simulink model "Quadrotor_model"  (R2020b)
settings: Solver=VariableStepAuto  StartTime=0.0  StopTime=10  RelTol=1e-3
model workspace (MAT data in the model file):
  Kheight = 1
  Kpitch = 1
  Kroll = 1
  Kyaw = 1
  pitch_dot_0 = 0
  roll_0 = 0
  roll_dot_0 = 0
  yaw_0 = 0
  yaw_dot_0 = 0
undefined symbols (not defined in the file or in its folder): pitch_0
libraries: pid_lib x4, simulink x1
settings Model: Creator=kike  LastModifiedBy=kike

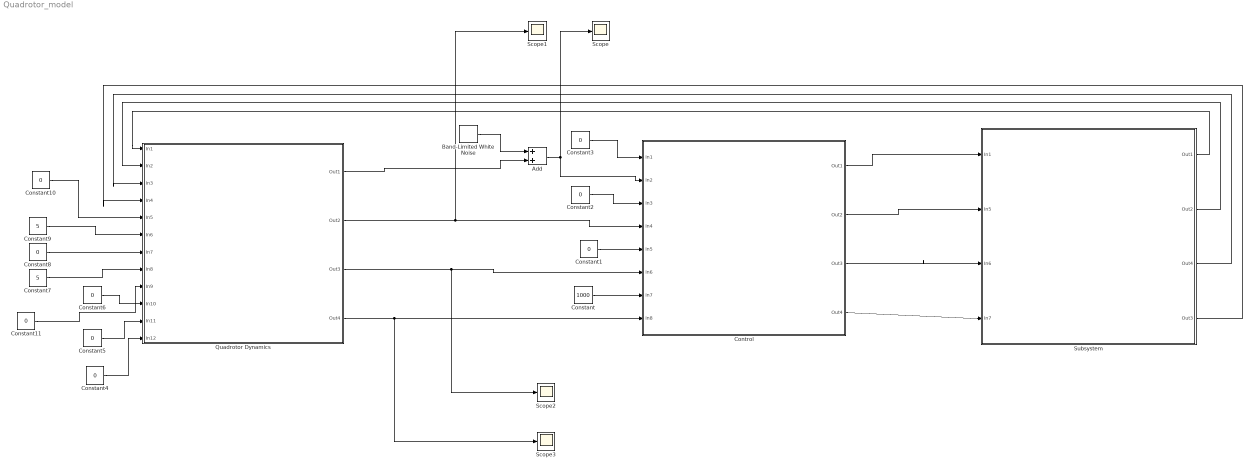
== system Quadrotor_model ==
  Add : Sum
  Band-Limited White Noise : simulink/Sources/Band-Limited White Noise  Cov=0  Ts=0.01  seed=[23341]
  Constant : Constant  Value=1000
  Constant{1..6,8,10..11} (9 alike) : Constant  Value=0
  Constant7 : Constant  Value=5
  Constant9 : Constant  Value=5
  Control : Subsystem
  Quadrotor Dynamics : Subsystem  Description=Quadrotor dynamics
  Scope{,1..3} (4 alike) : Scope
  Subsystem : Subsystem
  wires:
  Add/1 -> Scope/1, Control/2(In2)
  Quadrotor Dynamics/2(Out2) -> Scope1/1, Control/4(In4)
  Quadrotor Dynamics/3(Out3) -> Scope2/1, Control/6(In6)
  Quadrotor Dynamics/4(Out4) -> Scope3/1, Control/8(In8)
  Constant/1 -> Control/7(In7)
  Constant1/1 -> Control/5(In5)
  Constant2/1 -> Control/3(In3)
  Constant3/1 -> Control/1(In1)
  Constant4/1 -> Quadrotor Dynamics/12(In12)
  Constant5/1 -> Quadrotor Dynamics/11(In11)
  Constant6/1 -> Quadrotor Dynamics/10(In10)
  Constant7/1 -> Quadrotor Dynamics/8(In8)
  Constant8/1 -> Quadrotor Dynamics/7(In7)
  Constant9/1 -> Quadrotor Dynamics/6(In6)
  Constant10/1 -> Quadrotor Dynamics/5(In5)
  Constant11/1 -> Quadrotor Dynamics/9(In9)
  Control/1(Out1) -> Subsystem/1(In1)
  Control/2(Out2) -> Subsystem/2(In5)
  Control/3(Out3) -> Subsystem/3(In6)
  Control/4(Out4) -> Subsystem/4(In7)
  Subsystem/1(Out1) -> Quadrotor Dynamics/1(In1)
  Subsystem/2(Out2) -> Quadrotor Dynamics/2(In2)
  Subsystem/3(Out4) -> Quadrotor Dynamics/3(In3)
  Subsystem/4(Out3) -> Quadrotor Dynamics/4(In4)
  Band-Limited White Noise/1 -> Add/1
  Quadrotor Dynamics/1(Out1) -> Add/2

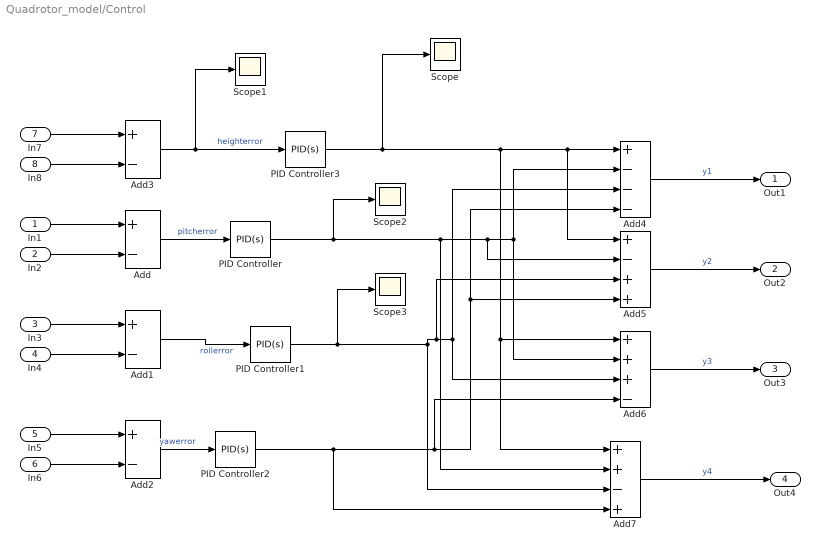
== system Quadrotor_model/Control ==
  In1 : Inport
  In2 : Inport  Port=2
  In3 : Inport  Port=3
  In4 : Inport  Port=4
  In5 : Inport  Port=5
  In6 : Inport  Port=6
  In7 : Inport  Port=7
  In8 : Inport  Port=8
  Add{,1..3} (4 alike) : Sum  Inputs=+-
  Add4 : Sum  Inputs=+---
  Add5 : Sum  Inputs=+-++
  Add6 : Sum  Inputs=+++-
  Add7 : Sum  Inputs=++-+
  PID Controller : pid_lib/PID Controller  Controller=PID  Form=Parallel  TimeDomain=Continuous-time  UseExternalTs=off  SampleTime=0.01  IntegratorMethod=Forward Euler  FilterMethod=Forward Euler  ControllerParametersSource=internal  P=10  I=0.5  D=10  UseFilter=on  N=100  TunerSelectOption=Transfer Function Based (PID Tuner App)  InitialConditionSource=internal  InitialConditionForIntegrator=0  InitialConditionForFilter=0  DifferentiatorICPrevScaledInput=0  ExternalReset=none  TrackingMode=off  Kt=1  LimitOutput=on  SatLimitsSource=internal  UpperSaturationLimit=100  LowerSaturationLimit=-100  LinearizeAsGain=on  AntiWindupMode=none  Kb=1  POutMin=[]  POutMax=[]  IOutMin=[]  IOutMax=[]  DOutMin=[]  DOutMax=[]  NOutMin=[]  NOutMax=[]  SumOutMin=[]  SumOutMax=[]  SaturationOutMin=[]  SaturationOutMax=[]  PParamMin=[]  PParamMax=[]  IParamMin=[]  IParamMax=[]  DParamMin=[]  DParamMax=[]  NParamMin=[]  NParamMax=[]  KbParamMin=[]  KbParamMax=[]  KtParamMin=[]  KtParamMax=[]  KbOutMin=[]  KbOutMax=[]  KtOutMin=[]  KtOutMax=[]  IntegratorOutMin=[]  IntegratorOutMax=[]  FilterOutMin=[]  FilterOutMax=[]  SumI1OutMin=[]  SumI1OutMax=[]  SumI2OutMin=[]  SumI2OutMax=[]  SumI3OutMin=[]  SumI3OutMax=[]  SumI4OutMin=[]  SumI4OutMax=[]  SumDOutMin=[]  SumDOutMax=[]  DifferentiatorOutMin=[]  DifferentiatorOutMax=[]  FilterDiffOutCoefMin=[]  FilterDiffOutCoefMax=[]  ReciprocalOutMin=[]  ReciprocalOutMax=[]  SumDenOutMin=[]  SumDenOutMax=[]  SumNumOutMin=[]  SumNumOutMax=[]  DivideOutMin=[]  DivideOutMax=[]  UdiffTsProdOutMin=[]  UdiffTsProdOutMax=[]  NTsProdOutMin=[]  NTsProdOutMax=[]  UintegralTsProdOutMin=[]  UintegralTsProdOutMax=[]  UngainTsProdOutMin=[]  UngainTsProdOutMax=[]  IntegratorContinuousStateAttributes=''  IntegratorStateMustResolveToSignalObject=off  IntegratorRTWStateStorageClass=Auto  FilterContinuousStateAttributes=''  FilterStateMustResolveToSignalObject=off  FilterRTWStateStorageClass=Auto  ParallelPVariant=InternalParameters  IdealPVariant=Disabled  IVariant=InternalParameters  DVariant=InternalParameters  IntegratorVariant=Continuous  SatVariant=Enabled  AWVariant=Passthrough  PCopyVariant=Disabled  TRVariant=Disabled  FdbkBlocksVariant=Forward  IdealPFdbkVariant=Disabled  SatFdbkVariant=Disabled  DerivativeFilterVariant=ContFilter  NVariant=InternalParameters  NCopyVariant=Disabled  FilterICVariant=InternalICsFilter  IntegratorICVariant=InternalICs  ExternalResetVariant=Disabled  TRSumVariant=Passthrough  SumFdbkVariant=Disabled  SumVariant=Sum_PID  TsampFilterVariant=InternalTs  TsampNgainVariant=Passthrough  TsampIntegralVariant=Passthrough  ExternalSaturationOutDataTypeStr=Inherit: Same as second input
  PID Controller1 : pid_lib/PID Controller  Controller=PID  Form=Parallel  TimeDomain=Continuous-time  UseExternalTs=off  SampleTime=-1  IntegratorMethod=Forward Euler  FilterMethod=Forward Euler  ControllerParametersSource=internal  P=10  I=0.5  D=10  UseFilter=on  N=100  TunerSelectOption=Transfer Function Based (PID Tuner App)  InitialConditionSource=internal  InitialConditionForIntegrator=0  InitialConditionForFilter=0  DifferentiatorICPrevScaledInput=0  ExternalReset=none  TrackingMode=off  Kt=1  LimitOutput=on  SatLimitsSource=internal  UpperSaturationLimit=100  LowerSaturationLimit=-100  LinearizeAsGain=on  AntiWindupMode=none  Kb=1  POutMin=[]  POutMax=[]  IOutMin=[]  IOutMax=[]  DOutMin=[]  DOutMax=[]  NOutMin=[]  NOutMax=[]  SumOutMin=[]  SumOutMax=[]  SaturationOutMin=[]  SaturationOutMax=[]  PParamMin=[]  PParamMax=[]  IParamMin=[]  IParamMax=[]  DParamMin=[]  DParamMax=[]  NParamMin=[]  NParamMax=[]  KbParamMin=[]  KbParamMax=[]  KtParamMin=[]  KtParamMax=[]  KbOutMin=[]  KbOutMax=[]  KtOutMin=[]  KtOutMax=[]  IntegratorOutMin=[]  IntegratorOutMax=[]  FilterOutMin=[]  FilterOutMax=[]  SumI1OutMin=[]  SumI1OutMax=[]  SumI2OutMin=[]  SumI2OutMax=[]  SumI3OutMin=[]  SumI3OutMax=[]  SumI4OutMin=[]  SumI4OutMax=[]  SumDOutMin=[]  SumDOutMax=[]  DifferentiatorOutMin=[]  DifferentiatorOutMax=[]  FilterDiffOutCoefMin=[]  FilterDiffOutCoefMax=[]  ReciprocalOutMin=[]  ReciprocalOutMax=[]  SumDenOutMin=[]  SumDenOutMax=[]  SumNumOutMin=[]  SumNumOutMax=[]  DivideOutMin=[]  DivideOutMax=[]  UdiffTsProdOutMin=[]  UdiffTsProdOutMax=[]  NTsProdOutMin=[]  NTsProdOutMax=[]  UintegralTsProdOutMin=[]  UintegralTsProdOutMax=[]  UngainTsProdOutMin=[]  UngainTsProdOutMax=[]  IntegratorContinuousStateAttributes=''  IntegratorStateMustResolveToSignalObject=off  IntegratorRTWStateStorageClass=Auto  FilterContinuousStateAttributes=''  FilterStateMustResolveToSignalObject=off  FilterRTWStateStorageClass=Auto  ParallelPVariant=InternalParameters  IdealPVariant=Disabled  IVariant=InternalParameters  DVariant=InternalParameters  IntegratorVariant=Continuous  SatVariant=Enabled  AWVariant=Passthrough  PCopyVariant=Disabled  TRVariant=Disabled  FdbkBlocksVariant=Forward  IdealPFdbkVariant=Disabled  SatFdbkVariant=Disabled  DerivativeFilterVariant=ContFilter  NVariant=InternalParameters  NCopyVariant=Disabled  FilterICVariant=InternalICsFilter  IntegratorICVariant=InternalICs  ExternalResetVariant=Disabled  TRSumVariant=Passthrough  SumFdbkVariant=Disabled  SumVariant=Sum_PID  TsampFilterVariant=InternalTs  TsampNgainVariant=Passthrough  TsampIntegralVariant=Passthrough  ExternalSaturationOutDataTypeStr=Inherit: Same as second input
  PID Controller2 : pid_lib/PID Controller  Controller=PID  Form=Parallel  TimeDomain=Continuous-time  UseExternalTs=off  SampleTime=-1  IntegratorMethod=Forward Euler  FilterMethod=Forward Euler  ControllerParametersSource=internal  P=0  I=0  D=0  UseFilter=on  N=100  TunerSelectOption=Transfer Function Based (PID Tuner App)  InitialConditionSource=internal  InitialConditionForIntegrator=0  InitialConditionForFilter=0  DifferentiatorICPrevScaledInput=0  ExternalReset=none  TrackingMode=off  Kt=1  LimitOutput=on  SatLimitsSource=internal  UpperSaturationLimit=100  LowerSaturationLimit=-100  LinearizeAsGain=on  AntiWindupMode=none  Kb=1  POutMin=[]  POutMax=[]  IOutMin=[]  IOutMax=[]  DOutMin=[]  DOutMax=[]  NOutMin=[]  NOutMax=[]  SumOutMin=[]  SumOutMax=[]  SaturationOutMin=[]  SaturationOutMax=[]  PParamMin=[]  PParamMax=[]  IParamMin=[]  IParamMax=[]  DParamMin=[]  DParamMax=[]  NParamMin=[]  NParamMax=[]  KbParamMin=[]  KbParamMax=[]  KtParamMin=[]  KtParamMax=[]  KbOutMin=[]  KbOutMax=[]  KtOutMin=[]  KtOutMax=[]  IntegratorOutMin=[]  IntegratorOutMax=[]  FilterOutMin=[]  FilterOutMax=[]  SumI1OutMin=[]  SumI1OutMax=[]  SumI2OutMin=[]  SumI2OutMax=[]  SumI3OutMin=[]  SumI3OutMax=[]  SumI4OutMin=[]  SumI4OutMax=[]  SumDOutMin=[]  SumDOutMax=[]  DifferentiatorOutMin=[]  DifferentiatorOutMax=[]  FilterDiffOutCoefMin=[]  FilterDiffOutCoefMax=[]  ReciprocalOutMin=[]  ReciprocalOutMax=[]  SumDenOutMin=[]  SumDenOutMax=[]  SumNumOutMin=[]  SumNumOutMax=[]  DivideOutMin=[]  DivideOutMax=[]  UdiffTsProdOutMin=[]  UdiffTsProdOutMax=[]  NTsProdOutMin=[]  NTsProdOutMax=[]  UintegralTsProdOutMin=[]  UintegralTsProdOutMax=[]  UngainTsProdOutMin=[]  UngainTsProdOutMax=[]  IntegratorContinuousStateAttributes=''  IntegratorStateMustResolveToSignalObject=off  IntegratorRTWStateStorageClass=Auto  FilterContinuousStateAttributes=''  FilterStateMustResolveToSignalObject=off  FilterRTWStateStorageClass=Auto  ParallelPVariant=InternalParameters  IdealPVariant=Disabled  IVariant=InternalParameters  DVariant=InternalParameters  IntegratorVariant=Continuous  SatVariant=Enabled  AWVariant=Passthrough  PCopyVariant=Disabled  TRVariant=Disabled  FdbkBlocksVariant=Forward  IdealPFdbkVariant=Disabled  SatFdbkVariant=Disabled  DerivativeFilterVariant=ContFilter  NVariant=InternalParameters  NCopyVariant=Disabled  FilterICVariant=InternalICsFilter  IntegratorICVariant=InternalICs  ExternalResetVariant=Disabled  TRSumVariant=Passthrough  SumFdbkVariant=Disabled  SumVariant=Sum_PID  TsampFilterVariant=InternalTs  TsampNgainVariant=Passthrough  TsampIntegralVariant=Passthrough  ExternalSaturationOutDataTypeStr=Inherit: Same as second input
  PID Controller3 : pid_lib/PID Controller  Controller=PID  Form=Parallel  TimeDomain=Continuous-time  UseExternalTs=off  SampleTime=-1  IntegratorMethod=Forward Euler  FilterMethod=Forward Euler  ControllerParametersSource=internal  P=2  I=1  D=2  UseFilter=on  N=100  TunerSelectOption=Transfer Function Based (PID Tuner App)  InitialConditionSource=internal  InitialConditionForIntegrator=0  InitialConditionForFilter=0  DifferentiatorICPrevScaledInput=0  ExternalReset=none  TrackingMode=off  Kt=1  LimitOutput=on  SatLimitsSource=internal  UpperSaturationLimit=800  LowerSaturationLimit=-800  LinearizeAsGain=on  AntiWindupMode=none  Kb=1  POutMin=[]  POutMax=[]  IOutMin=[]  IOutMax=[]  DOutMin=[]  DOutMax=[]  NOutMin=[]  NOutMax=[]  SumOutMin=[]  SumOutMax=[]  SaturationOutMin=[]  SaturationOutMax=[]  PParamMin=[]  PParamMax=[]  IParamMin=[]  IParamMax=[]  DParamMin=[]  DParamMax=[]  NParamMin=[]  NParamMax=[]  KbParamMin=[]  KbParamMax=[]  KtParamMin=[]  KtParamMax=[]  KbOutMin=[]  KbOutMax=[]  KtOutMin=[]  KtOutMax=[]  IntegratorOutMin=[]  IntegratorOutMax=[]  FilterOutMin=[]  FilterOutMax=[]  SumI1OutMin=[]  SumI1OutMax=[]  SumI2OutMin=[]  SumI2OutMax=[]  SumI3OutMin=[]  SumI3OutMax=[]  SumI4OutMin=[]  SumI4OutMax=[]  SumDOutMin=[]  SumDOutMax=[]  DifferentiatorOutMin=[]  DifferentiatorOutMax=[]  FilterDiffOutCoefMin=[]  FilterDiffOutCoefMax=[]  ReciprocalOutMin=[]  ReciprocalOutMax=[]  SumDenOutMin=[]  SumDenOutMax=[]  SumNumOutMin=[]  SumNumOutMax=[]  DivideOutMin=[]  DivideOutMax=[]  UdiffTsProdOutMin=[]  UdiffTsProdOutMax=[]  NTsProdOutMin=[]  NTsProdOutMax=[]  UintegralTsProdOutMin=[]  UintegralTsProdOutMax=[]  UngainTsProdOutMin=[]  UngainTsProdOutMax=[]  IntegratorContinuousStateAttributes=''  IntegratorStateMustResolveToSignalObject=off  IntegratorRTWStateStorageClass=Auto  FilterContinuousStateAttributes=''  FilterStateMustResolveToSignalObject=off  FilterRTWStateStorageClass=Auto  ParallelPVariant=InternalParameters  IdealPVariant=Disabled  IVariant=InternalParameters  DVariant=InternalParameters  IntegratorVariant=Continuous  SatVariant=Enabled  AWVariant=Passthrough  PCopyVariant=Disabled  TRVariant=Disabled  FdbkBlocksVariant=Forward  IdealPFdbkVariant=Disabled  SatFdbkVariant=Disabled  DerivativeFilterVariant=ContFilter  NVariant=InternalParameters  NCopyVariant=Disabled  FilterICVariant=InternalICsFilter  IntegratorICVariant=InternalICs  ExternalResetVariant=Disabled  TRSumVariant=Passthrough  SumFdbkVariant=Disabled  SumVariant=Sum_PID  TsampFilterVariant=InternalTs  TsampNgainVariant=Passthrough  TsampIntegralVariant=Passthrough  ExternalSaturationOutDataTypeStr=Inherit: Same as second input
  Scope{,1..3} (4 alike) : Scope
  Out1 : Outport
  Out2 : Outport  Port=2
  Out3 : Outport  Port=3
  Out4 : Outport  Port=4
  wires:
  In1/1 -> Add/1
  Add5/1 -> Out2/1  "y2"
  In4/1 -> Add1/2
  Add7/1 -> Out4/1  "y4"
  Add3/1 -> Scope1/1, PID Controller3/1  "heighterror"
  PID Controller1/1 -> Scope3/1, Add5/3, Add6/3, Add4/3, Add7/3
  PID Controller/1 -> Scope2/1, Add7/2, Add5/2, Add6/2, Add4/2
  Add/1 -> PID Controller/1  "pitcherror"
  PID Controller3/1 -> Scope/1, Add7/1, Add6/1, Add5/1, Add4/1
  In2/1 -> Add/2
  Add6/1 -> Out3/1  "y3"
  PID Controller2/1 -> Add7/4, Add6/4, Add5/4, Add4/4
  Add1/1 -> PID Controller1/1  "rollerror"
  In5/1 -> Add2/1
  In7/1 -> Add3/1
  In8/1 -> Add3/2
  Add2/1 -> PID Controller2/1  "yawerror"
  In6/1 -> Add2/2
  Add4/1 -> Out1/1  "y1"
  In3/1 -> Add1/1

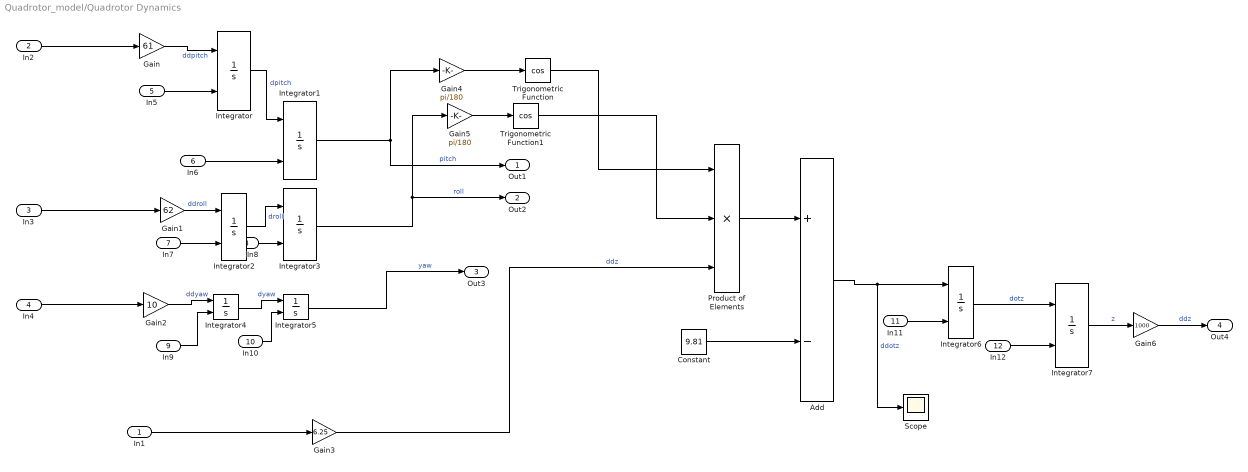
== system Quadrotor_model/Quadrotor Dynamics ==
  In1 : Inport
  In2 : Inport  Port=2
  In3 : Inport  Port=3
  In4 : Inport  Port=4
  In5 : Inport  Port=5
  In6 : Inport  Port=6
  In7 : Inport  Port=7
  In8 : Inport  Port=8
  In9 : Inport  Port=9
  In10 : Inport  Port=10
  In11 : Inport  Port=11
  In12 : Inport  Port=12
  Add : Sum  Inputs=+-
  Constant : Constant  Value=9.81
  Gain : Gain  Gain=61
  Gain1 : Gain  Gain=62
  Gain2 : Gain  Gain=10
  Gain3 : Gain  Gain=6.25
  Gain4 : Gain  Gain=pi/180
  Gain5 : Gain  Gain=pi/180
  Gain6 : Gain  Gain=1000
  Integrator : Integrator  InitialConditionSource=external  InitialCondition=pitch_dot_0
  Integrator1 : Integrator  InitialConditionSource=external  InitialCondition=pitch_0
  Integrator2 : Integrator  InitialConditionSource=external  InitialCondition=roll_dot_0
  Integrator3 : Integrator  InitialConditionSource=external  InitialCondition=roll_0
  Integrator4 : Integrator  InitialConditionSource=external  InitialCondition=yaw_dot_0
  Integrator5 : Integrator  InitialConditionSource=external
  Integrator6 : Integrator  InitialConditionSource=external  InitialCondition=yaw_dot_0
  Integrator7 : Integrator  InitialConditionSource=external  InitialCondition=yaw_dot_0
  Product of Elements : Product  Inputs=3
  Scope : Scope
  Trigonometric Function : Trigonometry  Operator=cos
  Trigonometric Function1 : Trigonometry  Operator=cos
  Out1 : Outport
  Out2 : Outport  Port=2
  Out3 : Outport  Port=3
  Out4 : Outport  Port=4
  wires:
  In8/1 -> Integrator3/2
  In9/1 -> Integrator4/2
  Product of Elements/1 -> Add/1
  In7/1 -> Integrator2/2
  In4/1 -> Gain2/1
  Gain2/1 -> Integrator4/1  "ddyaw"
  Trigonometric Function/1 -> Product of Elements/1
  In3/1 -> Gain1/1
  Constant/1 -> Add/2
  Gain1/1 -> Integrator2/1  "ddroll"
  Integrator4/1 -> Integrator5/1  "dyaw"
  Gain3/1 -> Product of Elements/3  "ddz"
  Integrator3/1 -> Out2/1, Gain5/1  "roll"
  Gain/1 -> Integrator/1  "ddpitch"
  In5/1 -> Integrator/2
  In6/1 -> Integrator1/2
  Integrator1/1 -> Out1/1, Gain4/1  "pitch"
  Integrator2/1 -> Integrator3/1  "droll"
  In2/1 -> Gain/1
  In10/1 -> Integrator5/2
  Integrator/1 -> Integrator1/1  "dpitch"
  Integrator5/1 -> Out3/1  "yaw"
  Integrator7/1 -> Gain6/1  "z"
  In11/1 -> Integrator6/2
  Integrator6/1 -> Integrator7/1  "dotz"
  Trigonometric Function1/1 -> Product of Elements/2
  In12/1 -> Integrator7/2
  In1/1 -> Gain3/1
  Add/1 -> Scope/1, Integrator6/1  "ddotz"
  Gain4/1 -> Trigonometric Function/1
  Gain5/1 -> Trigonometric Function1/1
  Gain6/1 -> Out4/1  "ddz"

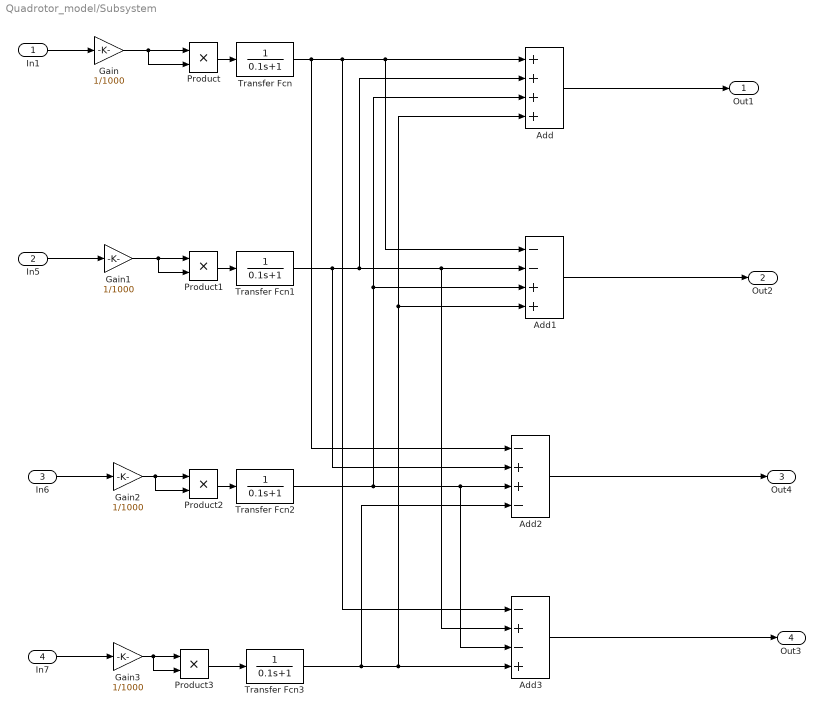
== system Quadrotor_model/Subsystem ==
  In1 : Inport
  In5 : Inport  Port=2
  In6 : Inport  Port=3
  In7 : Inport  Port=4
  Add : Sum  Inputs=++++
  Add1 : Sum  Inputs=--++
  Add2 : Sum  Inputs=-++-
  Add3 : Sum  Inputs=-+-+
  Gain{,1..3} (4 alike) : Gain  Gain=1/1000
  Product{,1..3} (4 alike) : Product
  Transfer Fcn{,1..3} (4 alike) : TransferFcn  Denominator=[0.1 1]
  Out1 : Outport
  Out2 : Outport  Port=2
  Out4 : Outport  Port=3
  Out3 : Outport  Port=4
  wires:
  In1/1 -> Gain/1
  In5/1 -> Gain1/1
  Add1/1 -> Out2/1
  Gain2/1 -> Product2/2, Product2/1
  Gain/1 -> Product/2, Product/1
  Add2/1 -> Out4/1
  Gain1/1 -> Product1/2, Product1/1
  Product2/1 -> Transfer Fcn2/1
  In7/1 -> Gain3/1
  Product/1 -> Transfer Fcn/1
  Product1/1 -> Transfer Fcn1/1
  In6/1 -> Gain2/1
  Product3/1 -> Transfer Fcn3/1
  Add/1 -> Out1/1
  Add3/1 -> Out3/1
  Gain3/1 -> Product3/2, Product3/1
  Transfer Fcn/1 -> Add2/1, Add3/1, Add/1, Add1/1
  Transfer Fcn1/1 -> Add2/2, Add/2, Add3/2, Add1/2
  Transfer Fcn2/1 -> Add3/3, Add2/3, Add1/3, Add/3
  Transfer Fcn3/1 -> Add2/4, Add3/4, Add1/4, Add/4
